simulink model "CPS_tare_Eva"  (R2022b)
settings: Solver=ode5  StartTime=0.0  StopTime=10.0  RelTol=1e-3
values from neighbouring files (symbols this model uses):
  T = 0.0002    [ringdown-circcyl-M10-d0_001-F1-workspace.mat]    (also in setup_CPS_parameters.m)
undefined symbols (not defined in the file or in its folder): National_Instruments, PCIe
libraries: sldrtlib x2, dspstat3 x1
settings Model: SimulationMode=external  Creator=eericks1  LastModifiedBy=eericks1
settings DataIOCC: ReturnWorkspaceOutputs=off
settings HardwareCC: ProdBitPerLong=64  ProdHWDeviceType=Intel->x86-64 (Linux 64)
settings RTWCC: Description=Simulink Desktop Real-Time  SystemTargetFile=sldrt.tlc  TemplateMakefile=sldrt.tmf  RTWCompilerOptimization=on
settings CodeAppCC: MaxIdLength=95
settings SimulinkDesktopRealTimeCC: TargetLibSuffix=_sldrt.a  TargetPreCompLibLocation=C:\Program Files\MATLAB\R2022b\toolbox\sldrt\lib\win64

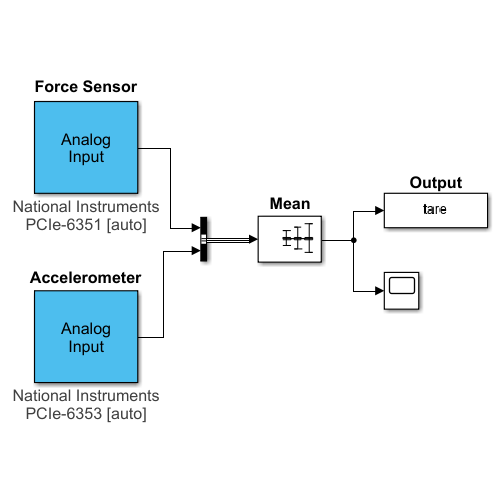
[thumbnail: Simulink's stored preview of the top-level diagram]
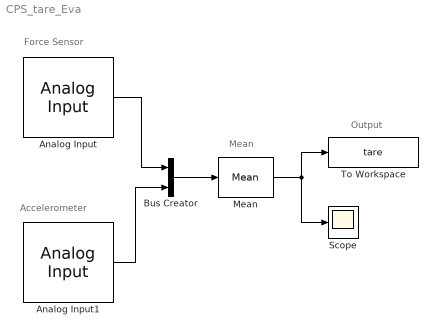
== system CPS_tare_Eva ==
  note: Accelerometer
  note: Mean
  note: Force Sensor
  note: Output
  Analog Input : sldrtlib/Analog Input  SampleTime=T  MaxMissedTicks=10  ShowMissedTicks=off  YieldWhenWaiting=off  DrvName=National_Instruments/PCIe-6351  DrvAddress=4294967295  DrvOptions=[1 0 0 0 0 0 0]  Channels=[1:6]  RangeMode=1  VoltRange=1  DataType=1
      settings: AttributesFormatString=National Instruments\nPCIe-6351 [auto]
  Analog Input1 : sldrtlib/Analog Input  SampleTime=T  MaxMissedTicks=10  ShowMissedTicks=off  YieldWhenWaiting=off  DrvName=National_Instruments/PCIe-6353  DrvAddress=4294967295  DrvOptions=[0 0 0 0 0 0 0]  Channels=[25]  RangeMode=1  VoltRange=1  DataType=1
      settings: AttributesFormatString=National Instruments\nPCIe-6353 [auto]
  Bus Creator : BusCreator  Inputs=2
  Mean : dspstat3/Mean  run=on  reset_popup=None  directionMode=Each column  dimension=1  roiEnable=off  roiType=Rectangles  roiPortion=Entire ROI  roiOutput=Individual statistics for each ROI  roiFlag=off  roundingMode=Floor  overflowMode=off  outputDataTypeStr=Inherit: Same as accumulator  outputMin=[]  outputMax=[]  outputLastDataTypeStr=Inherit: Same as accumulator
  Scope : Scope
  To Workspace : ToWorkspace  VariableName=tare  SaveFormat=Structure With Time  SampleTime=-1
  wires:
  Analog Input1/1 -> Bus Creator/2
  Mean/1 -> To Workspace/1, Scope/1
  Analog Input/1 -> Bus Creator/1
  Bus Creator/1 -> Mean/1
